simulink model "Snake_Robot1"  (R2022b)
settings: Solver=FixedStepAuto  StartTime=0.0  StopTime=100  FixedStep=0.001  RelTol=1e-3
undefined symbols (not defined in the file or in its folder): X, Y, Z
libraries: sm_lib x44, nesl_utility x21, slpidlib x3
(part 2 of 2)

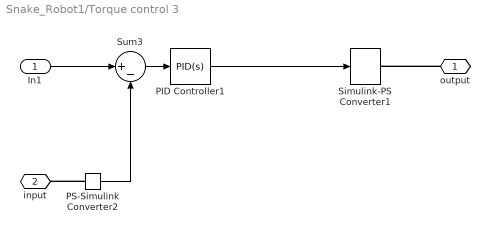
== system Snake_Robot1/Torque control 3 ==
  In1 : Inport
  PID Controller1 : slpidlib/PID Controller  Controller=PID  Form=Parallel  TimeDomain=Continuous-time  UseExternalTs=off  SampleTime=-1  IntegratorMethod=Forward Euler  FilterMethod=Forward Euler  ControllerParametersSource=internal  P=2  I=0.4  UseKiTs=off  D=0.05  N=1  UseFilter=on  TunerSelectOption=Transfer Function Based (PID Tuner App)  InitialConditionSource=internal  InitialConditionForIntegrator=0  InitialConditionForFilter=0  DifferentiatorICPrevScaledInput=0  ExternalReset=none  TrackingMode=off  Kt=1  LimitOutput=off  SatLimitsSource=internal  UpperSaturationLimit=inf  LowerSaturationLimit=-inf  LinearizeAsGain=on  AntiWindupMode=none  Kb=1  LimitIntegrator=off  UpperIntegratorSaturationLimit=inf  LowerIntegratorSaturationLimit=-inf  POutMin=[]  POutMax=[]  IOutMin=[]  IOutMax=[]  DOutMin=[]  DOutMax=[]  NOutMin=[]  NOutMax=[]  SumOutMin=[]  SumOutMax=[]  SaturationOutMin=[]  SaturationOutMax=[]  PParamMin=[]  PParamMax=[]  IParamMin=[]  IParamMax=[]  DParamMin=[]  DParamMax=[]  NParamMin=[]  NParamMax=[]  KbParamMin=[]  KbParamMax=[]  KtParamMin=[]  KtParamMax=[]  KbOutMin=[]  KbOutMax=[]  KtOutMin=[]  KtOutMax=[]  IntegratorOutMin=[]  IntegratorOutMax=[]  FilterOutMin=[]  FilterOutMax=[]  SumI1OutMin=[]  SumI1OutMax=[]  SumI2OutMin=[]  SumI2OutMax=[]  SumI3OutMin=[]  SumI3OutMax=[]  SumI4OutMin=[]  SumI4OutMax=[]  SumDOutMin=[]  SumDOutMax=[]  DifferentiatorOutMin=[]  DifferentiatorOutMax=[]  FilterDiffOutCoefMin=[]  FilterDiffOutCoefMax=[]  ReciprocalOutMin=[]  ReciprocalOutMax=[]  SumDenOutMin=[]  SumDenOutMax=[]  SumNumOutMin=[]  SumNumOutMax=[]  DivideOutMin=[]  DivideOutMax=[]  UdiffTsProdOutMin=[]  UdiffTsProdOutMax=[]  NTsProdOutMin=[]  NTsProdOutMax=[]  UintegralTsProdOutMin=[]  UintegralTsProdOutMax=[]  UngainTsProdOutMin=[]  UngainTsProdOutMax=[]  ClampingZeroOutDataTypeStr=Inherit: Inherit via back propagation  ClampingZeroOutMin=[]  ClampingZeroOutMax=[]  FilterDenConstantOutDataTypeStr=Inherit: Inherit via back propagation  FilterDenConstantOutMin=[]  FilterDenConstantOutMax=[]  PCopyOutDataTypeStr=Inherit: Inherit via back propagation  PCopyOutMin=[]  PCopyOutMax=[]  NCopyOutDataTypeStr=Inherit: Inherit via back propagation  NCopyOutMin=[]  NCopyOutMax=[]  IntegratorContinuousStateAttributes=''  IntegratorStateMustResolveToSignalObject=off  IntegratorRTWStateStorageClass=Auto  FilterContinuousStateAttributes=''  FilterStateMustResolveToSignalObject=off  FilterRTWStateStorageClass=Auto  ParallelPVariant=InternalParameters  IdealPVariant=Disabled  IVariant=InternalParameters  DVariant=InternalParameters  IntegratorVariant=Continuous  SatVariant=Disabled  AWVariant=Passthrough  PCopyVariant=Disabled  TRVariant=Disabled  FdbkBlocksVariant=Forward  IdealPFdbkVariant=Disabled  SatFdbkVariant=Disabled  DerivativeFilterVariant=ContFilter  NVariant=InternalParameters  NCopyVariant=Disabled  FilterICVariant=InternalICsFilter  IntegratorICVariant=InternalICs  ExternalResetVariant=Disabled  TRSumVariant=Passthrough  SumFdbkVariant=Disabled  SumVariant=Sum_PID  TsampFilterVariant=InternalTs  TsampNgainVariant=Passthrough  TsampIntegralVariant=Passthrough  ExternalSaturationOutDataTypeStr=Inherit: Same as second input
  PS-Simulink Converter2 : nesl_utility/PS-Simulink Converter  PhysicalDomain=network_engine_domain  SubClassName=ps_output  LeftPortType=input  RightPortType=output  PseudoPeriodic=off  Frequencies=[]  VectorFormat=1-D array  Unit=inherit  AffineConversion=off
  Simulink-PS Converter1 : nesl_utility/Simulink-PS Converter  PhysicalDomain=network_engine_domain  SubClassName=ps_input  LeftPortType=input  RightPortType=output  PseudoPeriodic=off  Frequencies=[]  NoiseDistribution=none  NoiseParameters=[]  Unit=N*m  AffineConversion=off  FilteringAndDerivatives=filter  SimscapeFilterOrder=2  InputFilterTimeConstant=0.001  UdotUserProvided=1
  Sum3 : Sum  Inputs=|+-
  output : PMIOPort  Side=Right
  input : PMIOPort  Port=2  Side=Left
  wires:
  PS-Simulink Converter2/1 -> Sum3/2
  Sum3/1 -> PID Controller1/1
  In1/1 -> Sum3/1
  PID Controller1/1 -> Simulink-PS Converter1/1
  connections:
  output/RConn1 -- Simulink-PS Converter1/RConn1
  PS-Simulink Converter2/LConn1 -- input/RConn1

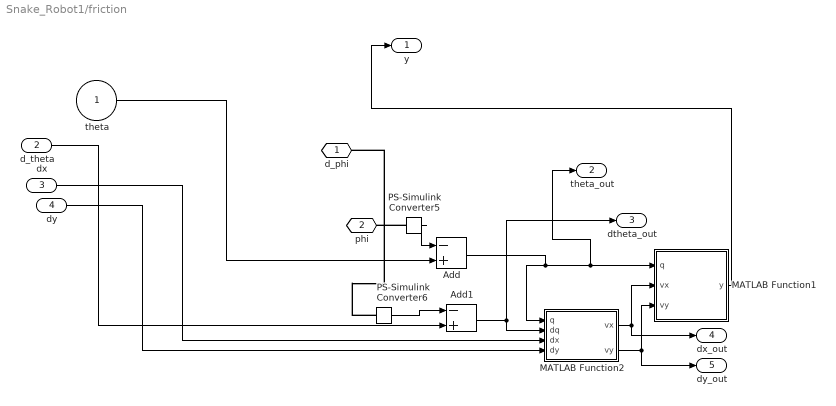
== system Snake_Robot1/friction ==
  theta : Inport
  d_theta : Inport  Port=2
  dx : Inport  Port=3
  dy : Inport  Port=4
  Add : Sum  Inputs=-+
  Add1 : Sum  Inputs=-+
  MATLAB Function1 : MATLAB Function  TreatAsAtomicUnit=on
  MATLAB Function2 : MATLAB Function  TreatAsAtomicUnit=on
  PS-Simulink Converter5 : nesl_utility/PS-Simulink Converter  PhysicalDomain=network_engine_domain  SubClassName=ps_output  LeftPortType=input  RightPortType=output  PseudoPeriodic=off  Frequencies=[]  VectorFormat=inherit  Unit=inherit  AffineConversion=off
  PS-Simulink Converter6 : nesl_utility/PS-Simulink Converter  PhysicalDomain=network_engine_domain  SubClassName=ps_output  LeftPortType=input  RightPortType=output  PseudoPeriodic=off  Frequencies=[]  VectorFormat=inherit  Unit=inherit  AffineConversion=off
  d_phi : PMIOPort  Side=Left
  phi : PMIOPort  Port=2  Side=Left
  y : Outport
  theta_out : Outport  Port=2
  dtheta_out : Outport  Port=3
  dx_out : Outport  Port=4
  dy_out : Outport  Port=5
  wires:
  MATLAB Function2/2(vy) -> dy_out/1, MATLAB Function1/3(vy)
  Add1/1 -> MATLAB Function2/2(dq), dtheta_out/1
  PS-Simulink Converter5/1 -> Add/1
  PS-Simulink Converter6/1 -> Add1/1
  MATLAB Function2/1(vx) -> MATLAB Function1/2(vx), dx_out/1
  dx/1 -> MATLAB Function2/3(dx)
  MATLAB Function1/1(y) -> y/1
  d_theta/1 -> Add1/2
  theta/1 -> Add/2
  dy/1 -> MATLAB Function2/4(dy)
  Add/1 -> MATLAB Function2/1(q), theta_out/1, MATLAB Function1/1(q)
  connections:
  PS-Simulink Converter5/LConn1 -- phi/RConn1
  PS-Simulink Converter6/LConn1 -- d_phi/RConn1

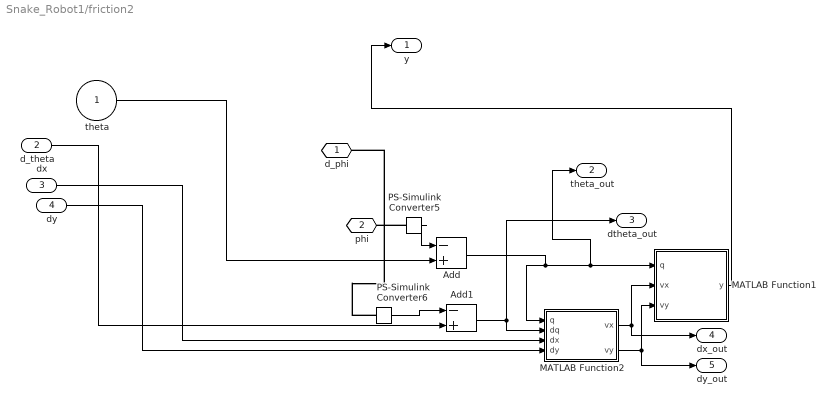
== system Snake_Robot1/friction2 ==
  theta : Inport
  d_theta : Inport  Port=2
  dx : Inport  Port=3
  dy : Inport  Port=4
  Add : Sum  Inputs=-+
  Add1 : Sum  Inputs=-+
  MATLAB Function1 : MATLAB Function  TreatAsAtomicUnit=on
  MATLAB Function2 : MATLAB Function  TreatAsAtomicUnit=on
  PS-Simulink Converter5 : nesl_utility/PS-Simulink Converter  PhysicalDomain=network_engine_domain  SubClassName=ps_output  LeftPortType=input  RightPortType=output  PseudoPeriodic=off  Frequencies=[]  VectorFormat=inherit  Unit=inherit  AffineConversion=off
  PS-Simulink Converter6 : nesl_utility/PS-Simulink Converter  PhysicalDomain=network_engine_domain  SubClassName=ps_output  LeftPortType=input  RightPortType=output  PseudoPeriodic=off  Frequencies=[]  VectorFormat=inherit  Unit=inherit  AffineConversion=off
  d_phi : PMIOPort  Side=Left
  phi : PMIOPort  Port=2  Side=Left
  y : Outport
  theta_out : Outport  Port=2
  dtheta_out : Outport  Port=3
  dx_out : Outport  Port=4
  dy_out : Outport  Port=5
  wires:
  MATLAB Function2/2(vy) -> dy_out/1, MATLAB Function1/3(vy)
  Add1/1 -> MATLAB Function2/2(dq), dtheta_out/1
  PS-Simulink Converter5/1 -> Add/1
  PS-Simulink Converter6/1 -> Add1/1
  MATLAB Function2/1(vx) -> MATLAB Function1/2(vx), dx_out/1
  dx/1 -> MATLAB Function2/3(dx)
  MATLAB Function1/1(y) -> y/1
  d_theta/1 -> Add1/2
  theta/1 -> Add/2
  dy/1 -> MATLAB Function2/4(dy)
  Add/1 -> MATLAB Function2/1(q), theta_out/1, MATLAB Function1/1(q)
  connections:
  PS-Simulink Converter5/LConn1 -- phi/RConn1
  PS-Simulink Converter6/LConn1 -- d_phi/RConn1

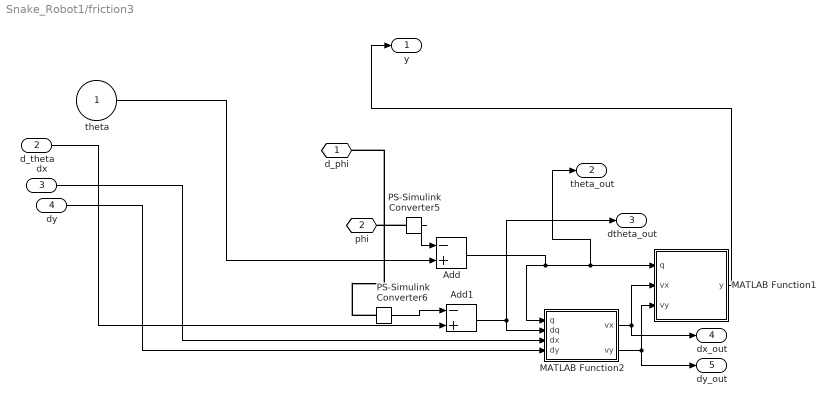
== system Snake_Robot1/friction3 ==
  theta : Inport
  d_theta : Inport  Port=2
  dx : Inport  Port=3
  dy : Inport  Port=4
  Add : Sum  Inputs=-+
  Add1 : Sum  Inputs=-+
  MATLAB Function1 : MATLAB Function  TreatAsAtomicUnit=on
  MATLAB Function2 : MATLAB Function  TreatAsAtomicUnit=on
  PS-Simulink Converter5 : nesl_utility/PS-Simulink Converter  PhysicalDomain=network_engine_domain  SubClassName=ps_output  LeftPortType=input  RightPortType=output  PseudoPeriodic=off  Frequencies=[]  VectorFormat=inherit  Unit=inherit  AffineConversion=off
  PS-Simulink Converter6 : nesl_utility/PS-Simulink Converter  PhysicalDomain=network_engine_domain  SubClassName=ps_output  LeftPortType=input  RightPortType=output  PseudoPeriodic=off  Frequencies=[]  VectorFormat=inherit  Unit=inherit  AffineConversion=off
  d_phi : PMIOPort  Side=Left
  phi : PMIOPort  Port=2  Side=Left
  y : Outport
  theta_out : Outport  Port=2
  dtheta_out : Outport  Port=3
  dx_out : Outport  Port=4
  dy_out : Outport  Port=5
  wires:
  Add/1 -> MATLAB Function1/1(q), theta_out/1, MATLAB Function2/1(q)
  dy/1 -> MATLAB Function2/4(dy)
  theta/1 -> Add/2
  d_theta/1 -> Add1/2
  MATLAB Function1/1(y) -> y/1
  dx/1 -> MATLAB Function2/3(dx)
  MATLAB Function2/1(vx) -> dx_out/1, MATLAB Function1/2(vx)
  PS-Simulink Converter6/1 -> Add1/1
  PS-Simulink Converter5/1 -> Add/1
  Add1/1 -> dtheta_out/1, MATLAB Function2/2(dq)
  MATLAB Function2/2(vy) -> MATLAB Function1/3(vy), dy_out/1
  connections:
  PS-Simulink Converter6/LConn1 -- d_phi/RConn1
  PS-Simulink Converter5/LConn1 -- phi/RConn1

== matlab function Snake_Robot1/friction/MATLAB Function1 ==
  data: q input; y output; vx input; vy input
function y = fcn(q,vx,vy)
ct =5;
cn = 10;
y = [ct*(cos(q))^2+cn*(sin(q))^2,(ct-cn)*sin(q)*cos(q);(ct-cn)*sin(q)*cos(q),ct*(sin(q))^2+cn*(cos(q))^2]*[vx;vy];

== matlab function Snake_Robot1/MATLAB Function ==
  data: q input; y output; vx input; vy input
function y = fcn(q,vx,vy)
ct =5;
cn = 10;
y = [ct*(cos(q))^2+cn*(sin(q))^2,(ct-cn)*sin(q)*cos(q);(ct-cn)*sin(q)*cos(q),ct*(sin(q))^2+cn*(cos(q))^2]*[vx;vy];

== matlab function Snake_Robot1/friction/MATLAB Function2 ==
  data: q input; vx output; dq input; dx input; dy input; vy output
function [vx,vy] = fcn(q,dq,dx,dy)
l =0.18;
vx=-l*sin(q)*dq - l*sin(q)*dq + dx;
vy= l*cos(q)*dq + l*cos(q)*dq + dy;

== matlab function Snake_Robot1/friction2/MATLAB Function1 ==
  data: q input; y output; vx input; vy input
function y = fcn(q,vx,vy)
ct = 5;
cn =10;
y = [ct*(cos(q))^2+cn*(sin(q))^2,(ct-cn)*sin(q)*cos(q);(ct-cn)*sin(q)*cos(q),ct*(sin(q))^2+cn*(cos(q))^2]*[vx;vy];

== matlab function Snake_Robot1/friction2/MATLAB Function2 ==
  data: q input; vx output; dq input; dx input; dy input; vy output
function [vx,vy] = fcn(q,dq,dx,dy)
l =0.18;
vx=-l*sin(q)*dq - l*sin(q)*dq + dx;
vy= l*cos(q)*dq + l*cos(q)*dq + dy;

== matlab function Snake_Robot1/friction3/MATLAB Function1 ==
  data: q input; y output; vx input; vy input
function y = fcn(q,vx,vy)
ct = 5;
cn = 10;
y = [ct*(cos(q))^2+cn*(sin(q))^2,(ct-cn)*sin(q)*cos(q);(ct-cn)*sin(q)*cos(q),ct*(sin(q))^2+cn*(cos(q))^2]*[vx;vy];

== matlab function Snake_Robot1/friction3/MATLAB Function2 ==
  data: q input; vx output; dq input; dx input; dy input; vy output
function [vx,vy] = fcn(q,dq,dx,dy)
l =0.18;
vx=-l*sin(q)*dq - l*sin(q)*dq + dx;
vy= l*cos(q)*dq + l*cos(q)*dq + dy;
